simulink model "baseline_queso_ground"  (R2021a)
settings: Solver=FixedStepAuto  StartTime=0.0  StopTime=50  FixedStep=framePeriod_s  RelTol=1e-3
undefined symbols (not defined in the file or in its folder): Aircraft, framePeriod_s
libraries: simulink x3
settings Model: Creator=brian  LastModifiedBy=Tuan Luong
settings SolverCC: AlgebraicLoopSolver=TrustRegion
settings OptimizationCC: DefaultParameterBehavior=Inlined  GainParamInheritBuiltInType=on  UseFloatMulNetSlope=on  DefaultUnderspecifiedDataType=single  InlineInvariantSignals=on  PassReuseOutputArgsAs=Individual arguments  ZeroExternalMemoryAtStartup=off  ZeroInternalMemoryAtStartup=off  NoFixptDivByZeroProtection=on  EfficientFloat2IntCast=on  LifeSpan=1  OptimizeBlockOrder=speed  DifferentSizesBufferReuse=on  EfficientTunableParamExpr=on
settings DebuggingCC: ParameterTunabilityLossMsg=error  SFMachineParentedDataDiag=warning
settings HardwareCC: ProdBitPerPointer=32  ProdBitPerSizeT=32  ProdBitPerPtrDiffT=32  ProdLargestAtomicInteger=Long  ProdLargestAtomicFloat=Double  ProdWordSize=32  ProdLongLongMode=on  ProdHWDeviceType=NXP->Cortex-M4
settings ModelReferenceCC: ModelReferenceNumInstancesAllowed=Single
settings SFSimCC: SimParseCustomCode=off  MATLABDynamicMemAlloc=off
settings RTWCC: SystemTargetFile=ert.tlc  GenCodeOnly=on  TemplateMakefile=ert_default_tmf  RTWVerbose=off  Toolchain=Microsoft Visual C++ 2019 v16.0 | nmake (64-bit Windows)  BuildConfiguration=Faster Runs  TargetLang=C++
settings CodeAppCC: ForceParamTrailComments=on  IgnoreCustomStorageClasses=off  OperatorAnnotations=on  SimulinkDataObjDesc=on  SFDataObjDesc=on  CustomSymbolStrGlobalVar=rt$N$M  CustomSymbolStrType=$N$M  CustomSymbolStrFcn=$N$M$F  CustomSymbolStrMacro=$N$M  InsertBlockDesc=on
settings ERTTargetCC: TargetLangStandard=C++03 (ISO)  IncludeMdlTerminateFcn=off  CombineSignalStateStructs=on  SuppressErrorStatus=on  SupportAbsoluteTime=off  CodeInterfacePackaging=C++ class  SupportComplex=off  ERTHeaderFileRootName=autocode$E  ERTSourceFileRootName=autocode$E  InlinedParameterPlacement=NonHierarchical  RootIOFormat=Structure reference  ERTCustomFileTemplate=example_file_process.tlc  ERTFilePackagingFormat=Compact  ArrayContainerType=std::array

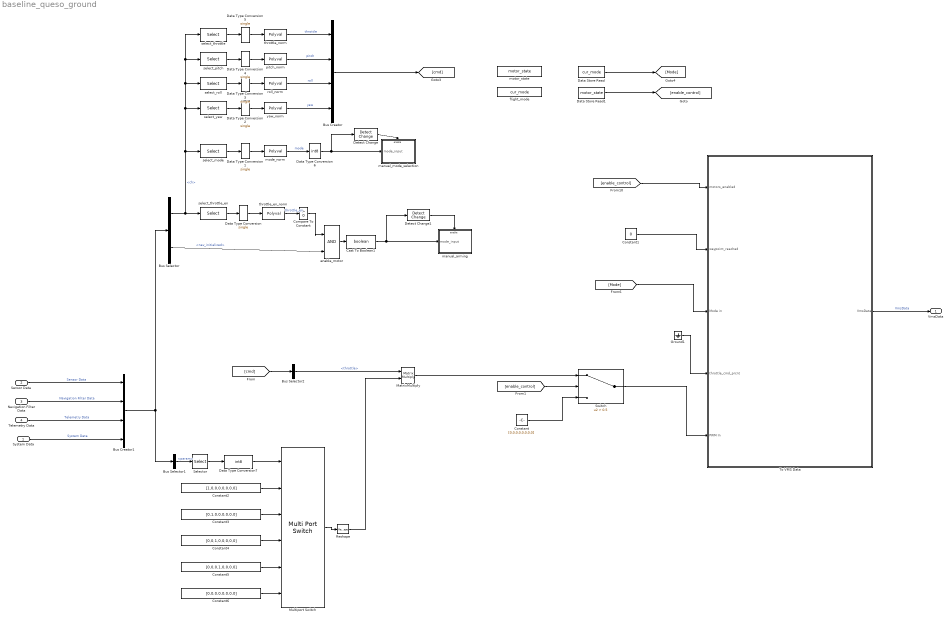
== system baseline_queso_ground ==
  System Data : Inport  OutDataTypeStr=Bus: SysData  SampleTime=framePeriod_s  BusOutputAsStruct=on
  Sensor Data : Inport  Port=2  OutDataTypeStr=Bus: SensorData  SampleTime=framePeriod_s  BusOutputAsStruct=on
  Navigation Filter Data : Inport  Port=3  OutDataTypeStr=Bus: NavData  SampleTime=framePeriod_s  BusOutputAsStruct=on
  Telemetry Data : Inport  Port=4  OutDataTypeStr=Bus: TelemData  SampleTime=framePeriod_s  BusOutputAsStruct=on
  Bus Creator : BusCreator  Inputs=4
  Bus Creator1 : BusCreator  Inputs=4
  Bus Selector : BusSelector  OutputSignals=Sensor Data.inceptor.ch,Navigation Filter Data.nav_initialized
  Bus Selector1 : BusSelector  OutputSignals=Telemetry Data.param
  Bus Selector2 : BusSelector  OutputSignals=throttle
  Cast To Boolean1 : DataTypeConversion  OutDataTypeStr=boolean
  Compare To Constant : simulink/Logic and Bit Operations/Compare To Constant  relop=>  const=0  OutDataTypeStr=boolean
  Constant : Constant  Value=[0,0,0,0,0,0,0,0]  OutDataTypeStr=single
  Constant1 : Constant  Value=0  OutDataTypeStr=boolean
  Constant2 : Constant  Value=[1,0,0,0,0,0,0,0]  OutDataTypeStr=single
  Constant3 : Constant  Value=[0,1,0,0,0,0,0,0]  OutDataTypeStr=single
  Constant4 : Constant  Value=[0,0,1,0,0,0,0,0]  OutDataTypeStr=single
  Constant5 : Constant  Value=[0,0,0,1,0,0,0,0]  OutDataTypeStr=single
  Constant6 : Constant  Value=[0,0,0,0,0,0,0,0]  OutDataTypeStr=single
  Data Store Read : DataStoreRead  DataStoreName=cur_mode  IndexOptions=Index vector (dialog)  Indices=1  OutputSizes=1
  Data Store Read1 : DataStoreRead  DataStoreName=motor_state  IndexOptions=Index vector (dialog)  Indices=1  OutputSizes=1
  Data Type Conversion{,1..5} (6 alike) : DataTypeConversion  OutDataTypeStr=single
  Data Type Conversion6 : DataTypeConversion  OutDataTypeStr=int8  RndMeth=Nearest
  Data Type Conversion7 : DataTypeConversion  OutDataTypeStr=int8
  Detect Change : simulink/Logic and Bit Operations/Detect Change  vinit=0  OutDataTypeStr=boolean
  Detect Change1 : simulink/Logic and Bit Operations/Detect Change  vinit=0  OutDataTypeStr=boolean
  Ground1 : Ground
  MatrixMultiply : Product  Multiplication=Matrix(*)
  Multiport Switch : MultiPortSwitch  DataPortOrder=Zero-based contiguous  Inputs=5  zeroidx=on
  Reshape : Reshape  OutputDimensionality=Row vector (2-D)
  Selector : Selector  IndexMode=Zero-based  IndexOptions=Index vector (dialog)  Indices=0  OutputSizes=1
  Switch : Switch  Criteria=u2 > Threshold  Threshold=0.5
  To VMS Data : Subsystem
  enable_motor : Logic  IconShape=distinctive  AllPortsSameDT=off  OutDataTypeStr=boolean
  flight_mode : DataStoreMemory  DataStoreName=cur_mode  ReadBeforeWriteMsg=warning  WriteAfterWriteMsg=warning  WriteAfterReadMsg=warning  ShowAdditionalParam=off  OutDataTypeStr=int8
  manual_arming : Subsystem
  manual_mode_selection : Subsystem
  mode_norm : Polyval  Coefs=Aircraft.Inceptor.coef_3
  motor_state : DataStoreMemory  DataStoreName=motor_state  ReadBeforeWriteMsg=warning  WriteAfterWriteMsg=warning  WriteAfterReadMsg=warning  ShowAdditionalParam=off  OutDataTypeStr=boolean
  pitch_norm : Polyval  Coefs=Aircraft.Inceptor.coef_2
  roll_norm : Polyval  Coefs=Aircraft.Inceptor.coef_2
  select_mode : Selector  IndexOptions=Index vector (dialog)  Indices=Aircraft.Inceptor.mode0  OutputSizes=1
  select_pitch : Selector  IndexOptions=Index vector (dialog)  Indices=Aircraft.Inceptor.pitch  OutputSizes=1
  select_roll : Selector  IndexOptions=Index vector (dialog)  Indices=Aircraft.Inceptor.roll  OutputSizes=1
  select_throttle : Selector  IndexOptions=Index vector (dialog)  Indices=Aircraft.Inceptor.throttle  OutputSizes=1
  select_throttle_en : Selector  IndexOptions=Index vector (dialog)  Indices=Aircraft.Inceptor.throttle_en  OutputSizes=1
  select_yaw : Selector  IndexOptions=Index vector (dialog)  Indices=Aircraft.Inceptor.yaw  OutputSizes=1
  throttle_en_norm : Polyval  Coefs=Aircraft.Inceptor.coef_2
  throttle_norm : Polyval  Coefs=Aircraft.Inceptor.coef_1
  yaw_norm : Polyval  Coefs=Aircraft.Inceptor.coef_2
  VmsData : Outport  OutDataTypeStr=Bus: VmsData  SampleTime=framePeriod_s  BusOutputAsStruct=on
  wires:
  Telemetry Data/1 -> Bus Creator1/3  "Telemetry Data"
  System Data/1 -> Bus Creator1/4  "System Data"
  Sensor Data/1 -> Bus Creator1/1  "Sensor Data"
  Navigation Filter Data/1 -> Bus Creator1/2  "Navigation Filter Data"
  To VMS Data/1(VmsData) -> VmsData/1  "VmsData"
  [Mode] -> To VMS Data/3(Mode in)
  Bus Selector/2 -> enable_motor/2  "<nav_initialized>"
  enable_motor/1 -> Cast To Boolean1/1
  Constant1/1 -> To VMS Data/2(waypoint_reached)
  [enable_control] -> To VMS Data/1(motors_enabled)
  Ground1/1 -> To VMS Data/4(throttle_cmd_prcnt)
  Bus Selector/1 -> select_throttle/1, select_pitch/1, select_roll/1, select_yaw/1, select_mode/1, select_throttle_en/1  "<ch>"
  select_throttle/1 -> Data Type Conversion5/1
  select_pitch/1 -> Data Type Conversion4/1
  select_roll/1 -> Data Type Conversion3/1
  select_yaw/1 -> Data Type Conversion2/1
  select_mode/1 -> Data Type Conversion1/1
  throttle_norm/1 -> Bus Creator/1  "throttle"
  pitch_norm/1 -> Bus Creator/2  "pitch"
  roll_norm/1 -> Bus Creator/3  "roll"
  yaw_norm/1 -> Bus Creator/4  "yaw"
  throttle_en_norm/1 -> Compare To Constant/1  "throttle_en"
  Compare To Constant/1 -> enable_motor/1
  Bus Creator/1 -> [cmd]
  select_throttle_en/1 -> Data Type Conversion/1
  Data Type Conversion/1 -> throttle_en_norm/1
  Data Type Conversion1/1 -> mode_norm/1
  Data Type Conversion2/1 -> yaw_norm/1
  Data Type Conversion3/1 -> roll_norm/1
  Data Type Conversion4/1 -> pitch_norm/1
  Data Type Conversion5/1 -> throttle_norm/1
  mode_norm/1 -> Data Type Conversion6/1  "mode"
  Data Store Read/1 -> [Mode]
  Data Type Conversion6/1 -> manual_mode_selection/1(mode_input), Detect Change/1
  Detect Change/1 -> manual_mode_selection/Enable
  Detect Change1/1 -> manual_arming/Enable
  Cast To Boolean1/1 -> manual_arming/1(mode_input), Detect Change1/1
  Data Store Read1/1 -> [enable_control]
  Bus Creator1/1 -> Bus Selector1/1, Bus Selector/1
  Bus Selector1/1 -> Selector/1  "<param>"
  Selector/1 -> Data Type Conversion7/1
  MatrixMultiply/1 -> Switch/1
  [enable_control] -> Switch/2
  Constant/1 -> Switch/3
  Data Type Conversion7/1 -> Multiport Switch/1
  Constant2/1 -> Multiport Switch/2
  Constant3/1 -> Multiport Switch/3
  Constant4/1 -> Multiport Switch/4
  Constant5/1 -> Multiport Switch/5
  Constant6/1 -> Multiport Switch/6
  [cmd] -> Bus Selector2/1
  Bus Selector2/1 -> MatrixMultiply/1  "<throttle>"
  Multiport Switch/1 -> Reshape/1
  Switch/1 -> To VMS Data/5(PWM In)
  Reshape/1 -> MatrixMultiply/2

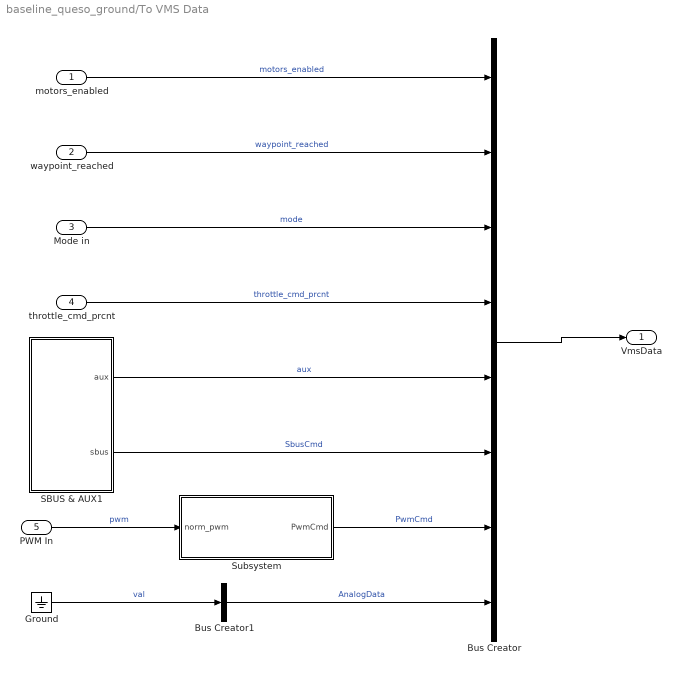
== system baseline_queso_ground/To VMS Data ==
  motors_enabled : Inport
  waypoint_reached : Inport  Port=2
  Mode in : Inport  Port=3
  throttle_cmd_prcnt : Inport  Port=4
  PWM In : Inport  Port=5
  Bus Creator : BusCreator  Inputs=8  OutDataTypeStr=Bus: VmsData  NonVirtualBus=on
  Bus Creator1 : BusCreator  Inputs=1  OutDataTypeStr=Bus: AnalogData
  Ground : Ground
  SBUS & AUX1 : Subsystem
  Subsystem : Subsystem
  VmsData : Outport
  wires:
  waypoint_reached/1 -> Bus Creator/2  "waypoint_reached"
  Mode in/1 -> Bus Creator/3  "mode"
  motors_enabled/1 -> Bus Creator/1  "motors_enabled"
  Bus Creator/1 -> VmsData/1
  throttle_cmd_prcnt/1 -> Bus Creator/4  "throttle_cmd_prcnt"
  PWM In/1 -> Subsystem/1(norm_pwm)  "pwm"
  Subsystem/1(PwmCmd) -> Bus Creator/7  "PwmCmd"
  SBUS & AUX1/1(aux) -> Bus Creator/5  "aux"
  SBUS & AUX1/2(sbus) -> Bus Creator/6  "SbusCmd"
  Bus Creator1/1 -> Bus Creator/8  "AnalogData"
  Ground/1 -> Bus Creator1/1  "val"

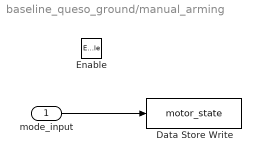
== system baseline_queso_ground/manual_arming ==
  mode_input : Inport
  Enable : EnablePort
  Data Store Write : DataStoreWrite  DataStoreName=motor_state  IndexOptions=Index vector (dialog)  Indices=1  OutputSizes=1
  wires:
  mode_input/1 -> Data Store Write/1

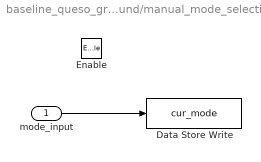
== system baseline_queso_ground/manual_mode_selection ==
  mode_input : Inport
  Enable : EnablePort
  Data Store Write : DataStoreWrite  DataStoreName=cur_mode  IndexOptions=Index vector (dialog)  Indices=1  OutputSizes=1
  wires:
  mode_input/1 -> Data Store Write/1

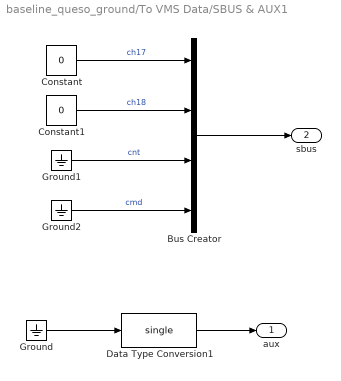
== system baseline_queso_ground/To VMS Data/SBUS & AUX1 ==
  Bus Creator : BusCreator  Inputs=4  OutDataTypeStr=Bus: SbusCmd  NonVirtualBus=on
  Constant : Constant  Value=0  OutDataTypeStr=boolean
  Constant1 : Constant  Value=0  OutDataTypeStr=boolean
  Data Type Conversion1 : DataTypeConversion  OutDataTypeStr=single
  Ground : Ground
  Ground1 : Ground
  Ground2 : Ground
  aux : Outport
  sbus : Outport  Port=2  SampleTime=framePeriod_s
  wires:
  Ground/1 -> Data Type Conversion1/1
  Data Type Conversion1/1 -> aux/1
  Bus Creator/1 -> sbus/1
  Constant/1 -> Bus Creator/1  "ch17"
  Constant1/1 -> Bus Creator/2  "ch18"
  Ground1/1 -> Bus Creator/3  "cnt"
  Ground2/1 -> Bus Creator/4  "cmd"

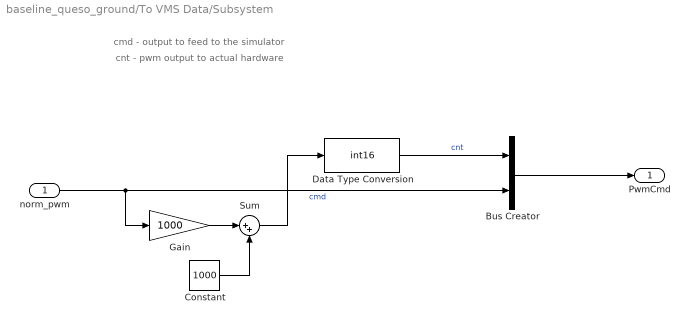
== system baseline_queso_ground/To VMS Data/Subsystem ==
  note: cmd - output to feed to the simulator
  note: cnt - pwm output to actual hardware
  norm_pwm : Inport
  Bus Creator : BusCreator  Inputs=2  OutDataTypeStr=Bus: PwmCmd  NonVirtualBus=on
      settings: InheritFromInputs=off
  Constant : Constant  Value=1000
  Data Type Conversion : DataTypeConversion  OutDataTypeStr=int16
  Gain : Gain  Gain=1000
  Sum : Sum  Inputs=|++
  PwmCmd : Outport
  wires:
  Constant/1 -> Sum/2
  Bus Creator/1 -> PwmCmd/1
  norm_pwm/1 -> Gain/1, Bus Creator/2  "cmd"
  Gain/1 -> Sum/1
  Sum/1 -> Data Type Conversion/1
  Data Type Conversion/1 -> Bus Creator/1  "cnt"
